simulink model "sf_debouncer"  (R2017b)
settings: Solver=VariableStepDiscrete  StartTime=0.0  StopTime=6  RelTol=1e-3  EnableMultiTasking=on
settings Model: Creator=The MathWorks, Inc.  LastModifiedBy=The MathWorks, Inc.
settings SolverCC: InsertRTBMode=Auto
settings DataIOCC: LimitDataPoints=on  SaveFormat=Array
settings OptimizationCC: ExpressionDepthLimit=2147483647  InitFltsAndDblsToZero=on  EfficientMapNaN2IntZero=off  LifeSpan=inf
settings DebuggingCC: SaveWithParameterizedLinksMsg=none  UnderspecifiedInitializationDetection=Classic  MergeDetectMultiDrivingBlocksExec=none  SignalResolutionControl=TryResolveAllWithWarning  SolverPrmCheckMsg=warning  MultiTaskDSMMsg=warning  MultiTaskCondExecSysMsg=none  FcnCallInpInsideContextMsg=warning  StateNameClashWarn=warning  StrictBusMsg=None  SFUnexpectedBacktrackingDiag=warning  SFNoUnconditionalDefaultTransitionDiag=warning  SFExecutionAtInitializationDiag=none
settings HardwareCC: ProdBitPerPointer=32  ProdBitPerSizeT=32  ProdBitPerPtrDiffT=32  ProdLargestAtomicFloat=None  ProdIntDivRoundTo=Undefined  ProdEndianess=Unspecified  ProdWordSize=32  ProdHWDeviceType=32-bit Generic
settings ModelReferenceCC: PropagateSignalLabelsOutOfModel=off
settings SFSimCC: SimParseCustomCode=off
settings CodeAppCC: StateflowObjectComments=on
settings GRTTargetCC: TargetFcnLib=ansi_tfl_tmw.mat  TargetLangStandard=C89/C90 (ANSI)  GeneratePreprocessorConditionals=Disable all  CombineOutputUpdateFcns=off  GRTInterface=on
settings ConfigComp: CovMetricSettings=dw  CovHtmlReporting=on  CovSaveCumulativeToWorkspaceVar=on  CovSaveSingleToWorkspaceVar=on  CovExternalEMLEnable=off  CovSFcnEnable=off

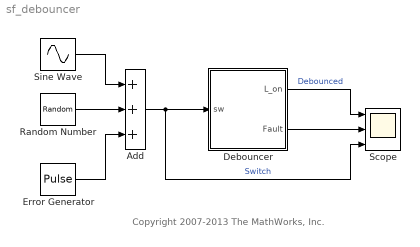
== system sf_debouncer ==
  note: Copyright 2007-2013 The MathWorks, Inc.
  Add : Sum  Inputs=+++
  Debouncer : Stateflow chart  TreatAsAtomicUnit=on
  Error Generator : DiscretePulseGenerator  PulseType=Time based  Amplitude=10  Period=0.001  PulseWidth=50  PhaseDelay=2
  Random Number : RandomNumber  Variance=30  SampleTime=0
  Scope : Scope  NumInputPorts=3
  Sine Wave : Sin  Amplitude=20  Frequency=10  SampleTime=0
  wires:
  Debouncer/1(L_on) -> Scope/1  "Debounced"
  Sine Wave/1 -> Add/1
  Random Number/1 -> Add/2
  Add/1 -> Debouncer/1(sw), Scope/3  "Switch"
  Error Generator/1 -> Add/3
  Debouncer/2(" Fault") -> Scope/2

== stateflow chart sf_debouncer/Debouncer ==
  settings: updateMethod=DISCRETE  sampleTime=0.001
  state Off
    en: L_on = 0;
    state Fault
      % Isolation
    state Normal
    Fault -> Normal : % Recovery
        | after(1, sec)
    (default) -> Normal
  state Debounce
    state Off
    state On
    Debounce.Off -> Debounce.On [order 2] : [sw > 0]
    Debounce.On -> Debounce.Off [order 2] : [sw < 0]
  state On
    en: L_on = 1;
  (default) -> Off
  Normal -> Debounce.On : [sw > 0]
  Debounce -> Fault : % Detection
      | after(0.3, sec)
  Debounce.Off -> Off [order 1] : after(0.1, sec)
  Debounce.On -> On [order 1] : after(0.1, sec)
  On -> Debounce.Off : [sw < 0]
  data: sw input; L_on output double; Fault output boolean
